simulink model "BlueBike"  (R2017b)
settings: Solver=VariableStepAuto  StartTime=0.0  StopTime=50  RelTol=1e-3
InitFcn:
  | INIT_BlueBike
undefined symbols (not defined in the file): b_contact_FW, b_contact_RW, C_F_alpha, C_F_kappa, CM_phi, Cylinder, Dtheta0, Dtheta0_FW, epsilon, g, isoCameraAimX, isoCameraX, isoCameraY, isoCameraZ, k_contact_FW, k_contact_RW, lengthFF, lengthFW, lengthRF, lengthRW, massFW, massRW, mB, mH, Parts_Lib, radiusFW, radiusRW, sigma, topViewY, topViewZ, X, xPla, Y, yPla, Z, zPla
libraries: sm_lib x75, nesl_utility x33, vrlib x14, dspsrcs4 x2, simulink x1
(part 4 of 4)

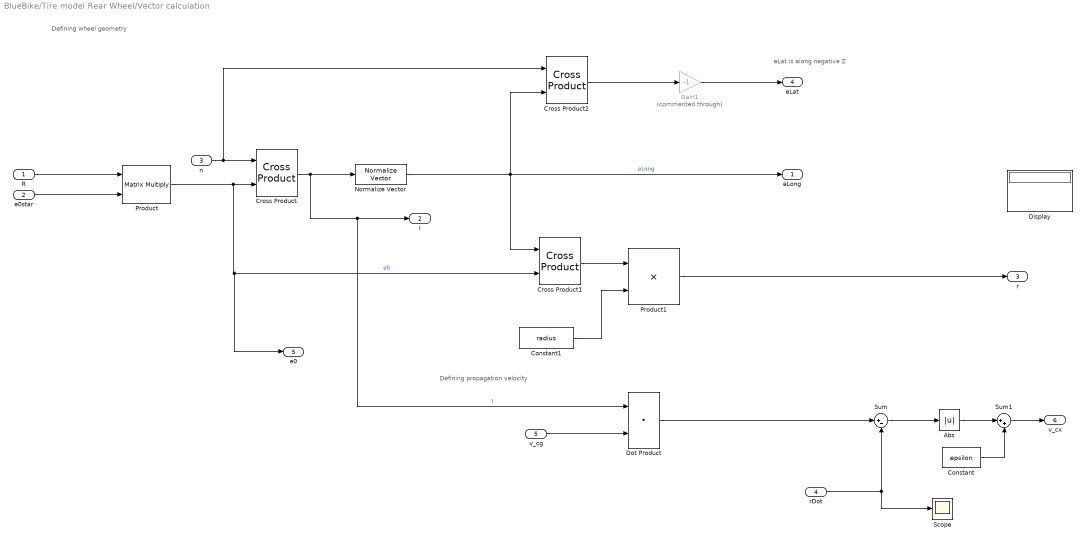
== system BlueBike/Tire model Rear Wheel/Vector calculation ==
  note: Defining propagation velocity
  note: Defining wheel geometry
  note: eLat is along
      | negative Z
  R : Inport
  e0star : Inport  Port=2
  n : Inport  Port=3
  rDot : Inport  Port=4
  v_cg : Inport  Port=5
  Abs : Abs  ZeroCross=off
  Constant : Constant  Value=epsilon
  Constant1 : Constant  Value=radius
  Cross Product : vrlib/Utilities/Cross Product
      settings: SourceProductBaseCode=VR
  Cross Product1 : vrlib/Utilities/Cross Product
      settings: SourceProductBaseCode=VR
  Cross Product2 : vrlib/Utilities/Cross Product
      settings: SourceProductBaseCode=VR
  Display : Display
  Dot Product : DotProduct  InputSameDT=on  OutDataTypeStr=Inherit: Inherit via internal rule
  Gain1 : Gain  Commented=through  Gain=-1
  Normalize Vector : vrlib/Utilities/Normalize Vector  maxzero=0
      settings: SourceProductName=Simulink 3D Animation  SourceProductBaseCode=VR
  Product : Product  Multiplication=Matrix(*)
  Product1 : Product
  Scope : Scope
  Sum : Sum  Inputs=|+-
  Sum1 : Sum  Inputs=|++
  eLong : Outport
  l : Outport  Port=2
  r : Outport  Port=3
  eLat : Outport  Port=4
  e0 : Outport  Port=5
  v_cx : Outport  Port=6
  wires:
  R/1 -> Product/1
  e0star/1 -> Product/2
  Product/1 -> Cross Product1/2, e0/1, Cross Product/2  "e0"
  n/1 -> Cross Product2/1, Cross Product/1
  Cross Product/1 -> Dot Product/1, l/1, Normalize Vector/1  "l"
  Normalize Vector/1 -> eLong/1, Cross Product2/2, Cross Product1/1  "eLong"
  Cross Product1/1 -> Product1/1
  Cross Product2/1 -> Gain1/1
  v_cg/1 -> Dot Product/2
  Dot Product/1 -> Sum/1
  Sum/1 -> Abs/1
  Abs/1 -> Sum1/1
  Sum1/1 -> v_cx/1
  Constant/1 -> Sum1/2
  Gain1/1 -> eLat/1
  Constant1/1 -> Product1/2
  rDot/1 -> Sum/2, Scope/1
  Product1/1 -> r/1

== system BlueBike/Tire model Rear Wheel/Verticle force ==
  x_cg : Inport
  v_s : Inport  Port=2
  r : Inport  Port=3
  n : Inport  Port=4
  Demux : Demux  Outputs=3
  Dot Product : DotProduct  InputSameDT=on  OutDataTypeStr=Inherit: Inherit via internal rule
  Dot Product1 : DotProduct  InputSameDT=on  OutDataTypeStr=Inherit: Inherit via internal rule
  Gain : Gain  Gain=-k_contact
  Gain1 : Gain  Gain=-b_contact
  Gain2 : Gain  Commented=through  Gain=-1
  Initial position of CP from ground : Constant  Value=[0 0 0]'
  Product : Product
  Scope : Scope
  Scope1 : Scope
  Sum : Sum  Inputs=|++
  Sum1 : Sum  Inputs=|+-
  Sum2 : Sum
  Fn : Outport
  FnDisk : Outport  Port=2
  wires:
  x_cg/1 -> Demux/1, Sum/1
  Sum/1 -> Sum1/1  "CP position from ground"
  Initial position of CP from ground/1 -> Sum1/2
  Sum1/1 -> Dot Product/1
  v_s/1 -> Dot Product1/2
  Dot Product1/1 -> Gain1/1  "pentration velocity"
  Sum2/1 -> Fn/1, Gain2/1, Scope1/1
  n/1 -> Product/2, Dot Product1/1, Dot Product/2
  r/1 -> Sum/2
  Gain2/1 -> Product/1
  Gain/1 -> Sum2/1
  Dot Product/1 -> Gain/1  "pen"
  Gain1/1 -> Sum2/2
  Product/1 -> FnDisk/1
  Demux/2 -> Scope/1

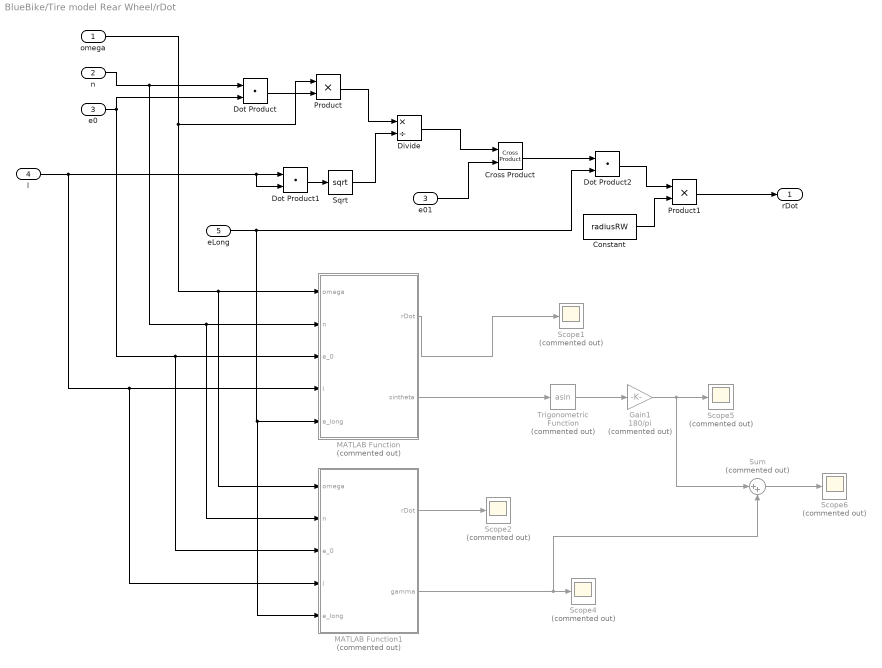
== system BlueBike/Tire model Rear Wheel/rDot ==
  omega : Inport
  n : Inport  Port=2
  e0 : Inport  Port=3
  l : Inport  Port=4
  eLong : Inport  Port=5
  Constant : Constant  Value=radiusRW
  Cross Product : vrlib/Utilities/Cross Product
      settings: SourceProductBaseCode=VR
  Divide : Product  Inputs=*/
  Dot Product : DotProduct  InputSameDT=on  OutDataTypeStr=Inherit: Inherit via internal rule
  Dot Product1 : DotProduct  InputSameDT=on  OutDataTypeStr=Inherit: Inherit via internal rule
  Dot Product2 : DotProduct  InputSameDT=on  OutDataTypeStr=Inherit: Inherit via internal rule
  Gain1 : Gain  Commented=on  Gain=180/pi
  MATLAB Function : MATLAB Function  Commented=on  TreatAsAtomicUnit=on
  MATLAB Function1 : MATLAB Function  Commented=on  TreatAsAtomicUnit=on
  Product : Product
  Product1 : Product
  Scope{1..2,4..6} (5 alike) : Scope  Commented=on
  Sqrt : Sqrt  SaturateOnIntegerOverflow=on
  Sum : Sum  Commented=on  Inputs=|++
  Trigonometric Function : Trigonometry  Commented=on  Operator=asin
  e01 : InportShadow  Port=3
  rDot : Outport
  wires:
  n/1 -> MATLAB Function1/2(n), MATLAB Function/2(n), Dot Product/1
  e0/1 -> MATLAB Function1/3(e_0), MATLAB Function/3(e_0), Dot Product/2
  Dot Product/1 -> Product/2
  omega/1 -> MATLAB Function1/1(omega), MATLAB Function/1(omega), Product/1
  Product/1 -> Divide/1
  l/1 -> MATLAB Function1/4(l), MATLAB Function/4(l), Dot Product1/2, Dot Product1/1
  Dot Product1/1 -> Sqrt/1
  Sqrt/1 -> Divide/2
  Divide/1 -> Cross Product/1
  e01/1 -> Cross Product/2
  Cross Product/1 -> Dot Product2/1
  eLong/1 -> MATLAB Function1/5(e_long), MATLAB Function/5(e_long), Dot Product2/2
  Dot Product2/1 -> Product1/1
  Constant/1 -> Product1/2
  MATLAB Function/1(rDot) -> Scope1/1
  MATLAB Function1/1(rDot) -> Scope2/1
  Product1/1 -> rDot/1
  MATLAB Function1/2(gamma) -> Sum/2, Scope4/1
  MATLAB Function/2(sintheta) -> Trigonometric Function/1
  Trigonometric Function/1 -> Gain1/1
  Gain1/1 -> Sum/1, Scope5/1
  Sum/1 -> Scope6/1

== matlab function BlueBike/Tire model Front Wheel/rDot/MATLAB Function1 ==
  data: rDot output; omega input; n input; e_0 input; l input; e_long input; gamma output
function [rDot,gamma] = fcn(omega,n,e_0,l,e_long)

sinGamma = dot(n,e_0);
firstTerm = (omega*sinGamma)/norm(l);
crossProd = cross(firstTerm,e_0);
rDot = dot(crossProd,e_long);
gamma = asind(sinGamma);

== matlab function BlueBike/Tire model Front Wheel/rDot/MATLAB Function ==
  data: rDot output; omega input; n input; e_0 input; l input; e_long input; radiusRW parameter; sintheta output
function [rDot,sintheta]  = fcn(omega,n,e_0,l,e_long, radiusRW)

sintheta = norm(l);
dotProd = dot(n,e_0);
firstTerm = omega * dotProd / sintheta;
crossProd = cross(firstTerm,e_0);
dotProd2 = dot(crossProd,e_long);
rDot = radiusRW * dotProd2;
% thetad = asind(sintheta) * (180/pi);

== matlab function BlueBike/Tire model Front Wheel/Slip model 2/MATLAB Function1 ==
  data: s1 input; s1 output
function s1 = fcn(s1)

if s1 < 1e-7 && s1 > -1e-7
    s1 = 0;
else
    s1 = s1;
end

== matlab function BlueBike/Tire model Front Wheel/Slip model 2/MATLAB Function2 ==
  data: s1 input; s1 output
function s1 = fcn(s1)

if s1 < 1e-8 && s1 > -1e-8
    s1 = 0;
else
    s1 = s1;
end

== matlab function BlueBike/Tire model Front Wheel/Longitudinal slip with relaxation/MATLAB Function2 ==
  data: s1 input; s1 output
function s1 = fcn(s1)

if s1 < 1e-15 && s1 > -1e-15
    s1 = 0;
else
    s1 = s1;
end

== matlab function BlueBike/Tire model Front Wheel/Lateral slip with relaxation/MATLAB Function2 ==
  data: s1 input; s1 output
function s1 = fcn(s1)

if s1 < 1e-3 && s1 > -1e-3
    s1 = 0;
else
    s1 = s1;
end

== matlab function BlueBike/Tire model Rear Wheel/Lateral slip with relaxation/MATLAB Function2 ==
  data: s1 input; s1 output
function s1 = fcn(s1)

if s1 < 1e-5 && s1 > -1e-5
    s1 = 0;
else
    s1 = s1;
end

== matlab function BlueBike/Tire model Rear Wheel/Longitudinal slip with relaxation/MATLAB Function2 ==
  data: s1 input; s1 output
function s1 = fcn(s1)

if s1 < 1e-5 && s1 > -1e-5
    s1 = 0;
else
    s1 = s1;
end

== matlab function BlueBike/Tire model Rear Wheel/Slip model 2/MATLAB Function1 ==
  data: s1 input; s1 output
function s1 = fcn(s1)

if s1 < 1e-7 && s1 > -1e-7
    s1 = 0;
else
    s1 = s1;
end

== matlab function BlueBike/Tire model Rear Wheel/Slip model 2/MATLAB Function2 ==
  data: s1 input; s1 output
function s1 = fcn(s1)

if s1 < 1e-8 && s1 > -1e-8
    s1 = 0;
else
    s1 = s1;
end

== matlab function BlueBike/Tire model Rear Wheel/rDot/MATLAB Function ==
  data: rDot output; omega input; n input; e_0 input; l input; e_long input; radiusRW parameter; sintheta output
function [rDot,sintheta]  = fcn(omega,n,e_0,l,e_long, radiusRW)

sintheta = norm(l);
dotProd = dot(n,e_0);
firstTerm = omega * dotProd / sintheta;
crossProd = cross(firstTerm,e_0);
dotProd2 = dot(crossProd,e_long);
rDot = radiusRW * dotProd2;
% thetad = asind(sintheta) * (180/pi);

== matlab function BlueBike/Tire model Rear Wheel/rDot/MATLAB Function1 ==
  data: rDot output; omega input; n input; e_0 input; l input; e_long input; gamma output
function [rDot,gamma] = fcn(omega,n,e_0,l,e_long)

sinGamma = dot(n,e_0);
firstTerm = (omega*sinGamma)/norm(l);
crossProd = cross(firstTerm,e_0);
rDot = dot(crossProd,e_long);
gamma = asind(sinGamma);
